simulink subsystem "Control_Attitude_Thrust"  (R2025b)
settings: Solver=VariableStepAuto  StartTime=0.0  StopTime=10.0  RelTol=1e-3
undefined symbols (not defined in the file): StabTrimPos
settings Model: Creator=invrt  LastModifiedBy=invrt

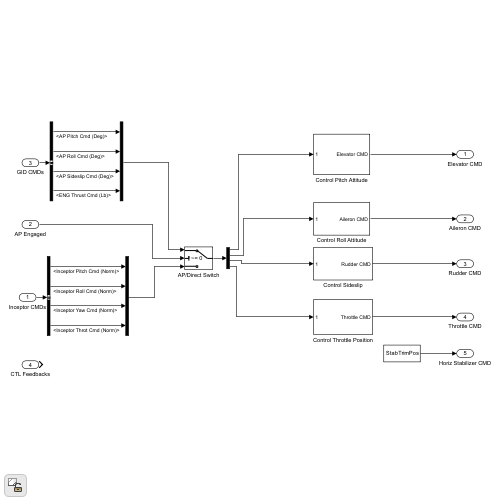
[thumbnail: Simulink's stored preview of the top-level diagram]
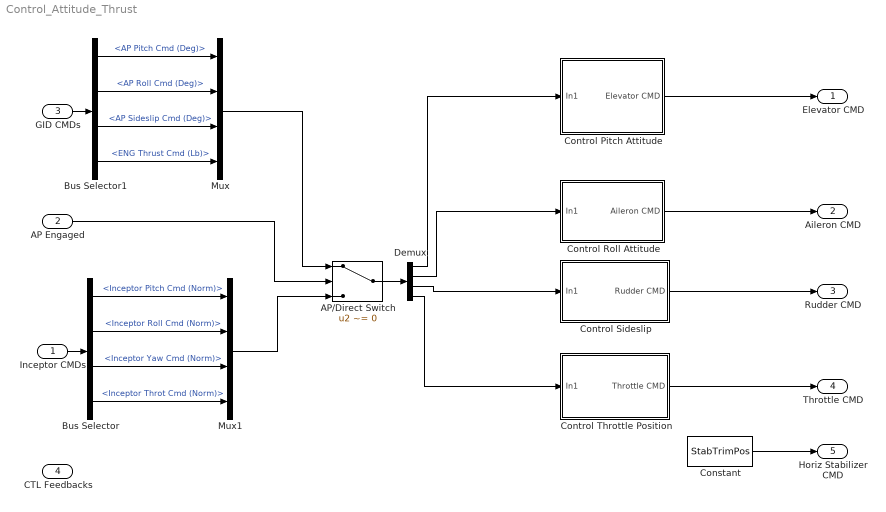
== system Control_Attitude_Thrust ==
  Inceptor CMDs : Inport
  AP Engaged : Inport  Port=2
  GID CMDs : Inport  Port=3
  CTL Feedbacks : Inport  Port=4
  AP/Direct Switch : Switch  Criteria=u2 ~= 0  SaturateOnIntegerOverflow=off  InputSameDT=off
  Bus Selector : BusSelector  OutputSignals=Inceptor Pitch Cmd (Norm),Inceptor Roll Cmd (Norm),Inceptor Yaw Cmd (Norm),Inceptor Throt Cmd (Norm)
  Bus Selector1 : BusSelector  OutputSignals=AP Pitch Cmd (Deg),AP Roll Cmd (Deg),AP Sideslip Cmd (Deg),ENG Thrust Cmd (Lb)
  Constant : Constant  Value=StabTrimPos
  Control Pitch Attitude : Subsystem
  Control Roll Attitude : Subsystem
  Control Sideslip : Subsystem
  Control Throttle Position : Subsystem
  Demux : Demux
  Mux : Mux
  Mux1 : Mux
  Elevator CMD : Outport
  Aileron CMD : Outport  Port=2
  Rudder CMD : Outport  Port=3
  Throttle CMD : Outport  Port=4
  Horiz Stabilizer CMD : Outport  Port=5
  wires:
  Inceptor CMDs/1 -> Bus Selector/1
  Bus Selector/1 -> Mux1/1  "<Inceptor Pitch Cmd (Norm)>"
  GID CMDs/1 -> Bus Selector1/1
  Bus Selector1/4 -> Mux/4  "<ENG Thrust Cmd (Lb)>"
  Bus Selector/2 -> Mux1/2  "<Inceptor Roll Cmd (Norm)>"
  Bus Selector1/2 -> Mux/2  "<AP Roll Cmd (Deg)>"
  Bus Selector1/1 -> Mux/1  "<AP Pitch Cmd (Deg)>"
  Bus Selector1/3 -> Mux/3  "<AP Sideslip Cmd (Deg)>"
  Bus Selector/3 -> Mux1/3  "<Inceptor Yaw Cmd (Norm)>"
  Bus Selector/4 -> Mux1/4  "<Inceptor Throt Cmd (Norm)>"
  Mux/1 -> AP/Direct Switch/1
  AP Engaged/1 -> AP/Direct Switch/2
  Mux1/1 -> AP/Direct Switch/3
  AP/Direct Switch/1 -> Demux/1
  Demux/1 -> Control Pitch Attitude/1(In1)
  Demux/2 -> Control Roll Attitude/1(In1)
  Demux/3 -> Control Sideslip/1(In1)
  Demux/4 -> Control Throttle Position/1(In1)
  Control Pitch Attitude/1(Elevator CMD) -> Elevator CMD/1
  Control Roll Attitude/1(Aileron CMD) -> Aileron CMD/1
  Control Throttle Position/1(Throttle CMD) -> Throttle CMD/1
  Control Sideslip/1(Rudder CMD) -> Rudder CMD/1
  Constant/1 -> Horiz Stabilizer CMD/1

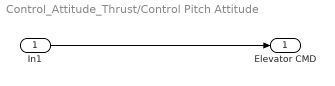
== system Control_Attitude_Thrust/Control Pitch Attitude ==
  In1 : Inport
  Elevator CMD : Outport
  wires:
  In1/1 -> Elevator CMD/1

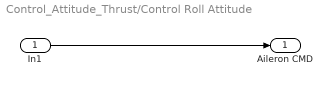
== system Control_Attitude_Thrust/Control Roll Attitude ==
  In1 : Inport
  Aileron CMD : Outport
  wires:
  In1/1 -> Aileron CMD/1

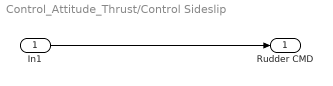
== system Control_Attitude_Thrust/Control Sideslip ==
  In1 : Inport
  Rudder CMD : Outport
  wires:
  In1/1 -> Rudder CMD/1

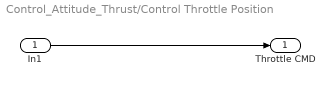
== system Control_Attitude_Thrust/Control Throttle Position ==
  In1 : Inport
  Throttle CMD : Outport
  wires:
  In1/1 -> Throttle CMD/1
